simulink model "PID_IdleSpeed"  (R2023b)
settings: Solver=ode15s  StartTime=0.0  StopTime=10  RelTol=1e-3
values from neighbouring files (symbols this model uses):
  DUM = cell2mat(DUM)    [PID_IdleSpeedCode.m]
  NUM = cell2mat(NUM)    [PID_IdleSpeedCode.m]
  Ts = 0.0001    [PID_RL_Tuner.m]
undefined symbols (not defined in the file or in its folder): DiscIntNeverNeededParam
libraries: deeplib x3, slpidlib x2, rllib x2, simulink x2
settings Model: Creator=mrmal  LastModifiedBy=rabia
settings SolverCC: AlgebraicLoopSolver=TrustRegion
settings DebuggingCC: UnconnectedInputMsg=warning  UnconnectedOutputMsg=warning  UnconnectedLineMsg=warning
settings ModelReferenceCC: EnableRefExpFcnMdlSchedulingChecks=on

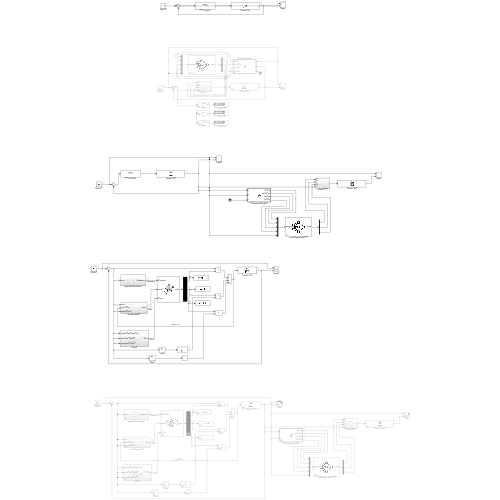
[thumbnail: Simulink's stored preview of the top-level diagram]
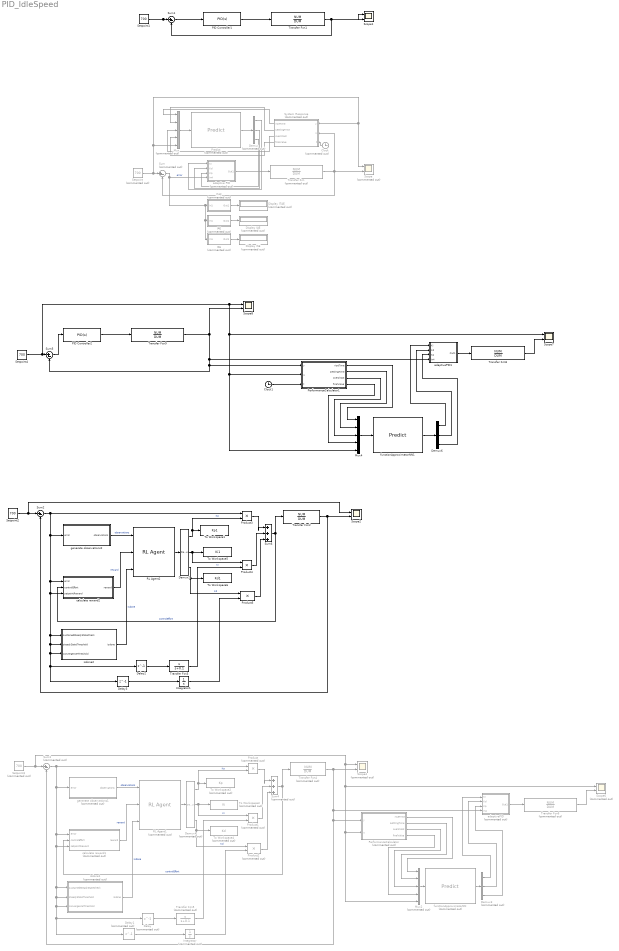
== system PID_IdleSpeed ==
  Clock : Clock  Commented=on
  Clock1 : Clock
  Delay : Delay  Commented=on  DelayLength=1  InitialCondition=0
  Delay1 : Delay  Commented=on  DelayLength=1  InitialCondition=0
  Delay2 : Delay  DelayLength=1  InitialCondition=0
  Delay3 : Delay  DelayLength=1  InitialCondition=0
  Demux : Demux  Commented=on  Outputs=3
  Demux2 : Demux  Outputs=3
  Demux3 : Demux  Commented=on  Outputs=3
  Demux4 : Demux  Commented=on  Outputs=3
  Demux6 : Demux  Outputs=3
  Display IAE : Display  Commented=on
  Display ISE : Display  Commented=on
  Display ITAE : Display  Commented=on
  IAE : Subsystem  Commented=on
      mask help:
      | IAE performacne index
      |
      | output = int |input| dt
      mask Display:
      | disp('IAE')
      | port_label('input',1,'e')
      | port_label('output',1,'iae')
  ISE : Subsystem  Commented=on
      mask help:
      | ISE performance index
      |
      | output = int (input)^2 dt
      mask Display:
      | disp('ISE')
      | port_label('input',1,'e')
      | port_label('output',1,'ise')
  ITAE : Subsystem  Commented=on
      mask help:
      | ITAE performance index
      |
      | output = int t|input| dt
      mask Display:
      | disp('ITAE')
      | port_label('input',1,'e')
      | port_label('output',1,'itae')
  Integrator : Integrator  Commented=on
  Integrator1 : Integrator
  Mux : Mux  Commented=on  Inputs=5
  Mux2 : Mux  Commented=on  Inputs=5
  Mux4 : Mux  Inputs=5
  PID Controller1 : slpidlib/PID Controller  Controller=PID  Form=Parallel  TimeDomain=Continuous-time  UseExternalTs=off  SampleTime=-1  IntegratorMethod=Forward Euler  FilterMethod=Forward Euler  ControllerParametersSource=internal  P=0.1  I=1  UseKiTs=off  D=0.001  N=54.2037558026899  UseFilter=on  TunerSelectOption=Transfer Function Based (PID Tuner App)  InitialConditionSource=internal  InitialConditionForIntegrator=0  InitialConditionForFilter=0  DifferentiatorICPrevScaledInput=0  ExternalReset=none  TrackingMode=off  Kt=1  LimitOutput=off  SatLimitsSource=internal  UpperSaturationLimit=inf  LowerSaturationLimit=-inf  LinearizeAsGain=on  AntiWindupMode=none  Kb=1  LimitIntegrator=off  UpperIntegratorSaturationLimit=inf  LowerIntegratorSaturationLimit=-inf  POutMin=[]  POutMax=[]  IOutMin=[]  IOutMax=[]  DOutMin=[]  DOutMax=[]  NOutMin=[]  NOutMax=[]  SumOutMin=[]  SumOutMax=[]  SaturationOutMin=[]  SaturationOutMax=[]  PParamMin=[]  PParamMax=[]  IParamMin=[]  IParamMax=[]  DParamMin=[]  DParamMax=[]  NParamMin=[]  NParamMax=[]  KbParamMin=[]  KbParamMax=[]  KtParamMin=[]  KtParamMax=[]  KbOutMin=[]  KbOutMax=[]  KtOutMin=[]  KtOutMax=[]  IntegratorOutMin=[]  IntegratorOutMax=[]  FilterOutMin=[]  FilterOutMax=[]  SumI1OutMin=[]  SumI1OutMax=[]  SumI2OutMin=[]  SumI2OutMax=[]  SumI3OutMin=[]  SumI3OutMax=[]  SumI4OutMin=[]  SumI4OutMax=[]  SumDOutMin=[]  SumDOutMax=[]  DifferentiatorOutMin=[]  DifferentiatorOutMax=[]  FilterDiffOutCoefMin=[]  FilterDiffOutCoefMax=[]  ReciprocalOutMin=[]  ReciprocalOutMax=[]  SumDenOutMin=[]  SumDenOutMax=[]  SumNumOutMin=[]  SumNumOutMax=[]  DivideOutMin=[]  DivideOutMax=[]  UdiffTsProdOutMin=[]  UdiffTsProdOutMax=[]  NTsProdOutMin=[]  NTsProdOutMax=[]  UintegralTsProdOutMin=[]  UintegralTsProdOutMax=[]  UngainTsProdOutMin=[]  UngainTsProdOutMax=[]  ClampingZeroOutDataTypeStr=Inherit: Inherit via back propagation  ClampingZeroOutMin=[]  ClampingZeroOutMax=[]  FilterDenConstantOutDataTypeStr=Inherit: Inherit via back propagation  FilterDenConstantOutMin=[]  FilterDenConstantOutMax=[]  PCopyOutDataTypeStr=Inherit: Inherit via back propagation  PCopyOutMin=[]  PCopyOutMax=[]  NCopyOutDataTypeStr=Inherit: Inherit via back propagation  NCopyOutMin=[]  NCopyOutMax=[]  IntegratorContinuousStateAttributes=''  IntegratorStateMustResolveToSignalObject=off  IntegratorRTWStateStorageClass=Auto  FilterContinuousStateAttributes=''  FilterStateMustResolveToSignalObject=off  FilterRTWStateStorageClass=Auto  ParallelPVariant=InternalParameters  IdealPVariant=Disabled  IVariant=InternalParameters  DVariant=InternalParameters  IntegratorVariant=Continuous  SatVariant=Disabled  AWVariant=Passthrough  PCopyVariant=Disabled  TRVariant=Disabled  FdbkBlocksVariant=Forward  IdealPFdbkVariant=Disabled  SatFdbkVariant=Disabled  DerivativeFilterVariant=ContFilter  NVariant=InternalParameters  NCopyVariant=Disabled  FilterICVariant=InternalICsFilter  IntegratorICVariant=InternalICs  ExternalResetVariant=Disabled  TRSumVariant=Passthrough  SumFdbkVariant=Disabled  SumVariant=Sum_PID  TsampFilterVariant=InternalTs  TsampNgainVariant=Passthrough  TsampIntegralVariant=Disabled_SignalSpec  ExternalSaturationOutDataTypeStr=Inherit: Same as second input
  PID Controller2 : slpidlib/PID Controller  Controller=PID  Form=Parallel  TimeDomain=Continuous-time  UseExternalTs=off  SampleTime=-1  IntegratorMethod=Forward Euler  FilterMethod=Forward Euler  ControllerParametersSource=internal  P=0.1  I=1  UseKiTs=off  D=0.001  N=54.2037558026899  UseFilter=on  TunerSelectOption=Transfer Function Based (PID Tuner App)  InitialConditionSource=internal  InitialConditionForIntegrator=0  InitialConditionForFilter=0  DifferentiatorICPrevScaledInput=0  ExternalReset=none  TrackingMode=off  Kt=1  LimitOutput=off  SatLimitsSource=internal  UpperSaturationLimit=inf  LowerSaturationLimit=-inf  LinearizeAsGain=on  AntiWindupMode=none  Kb=1  LimitIntegrator=off  UpperIntegratorSaturationLimit=inf  LowerIntegratorSaturationLimit=-inf  POutMin=[]  POutMax=[]  IOutMin=[]  IOutMax=[]  DOutMin=[]  DOutMax=[]  NOutMin=[]  NOutMax=[]  SumOutMin=[]  SumOutMax=[]  SaturationOutMin=[]  SaturationOutMax=[]  PParamMin=[]  PParamMax=[]  IParamMin=[]  IParamMax=[]  DParamMin=[]  DParamMax=[]  NParamMin=[]  NParamMax=[]  KbParamMin=[]  KbParamMax=[]  KtParamMin=[]  KtParamMax=[]  KbOutMin=[]  KbOutMax=[]  KtOutMin=[]  KtOutMax=[]  IntegratorOutMin=[]  IntegratorOutMax=[]  FilterOutMin=[]  FilterOutMax=[]  SumI1OutMin=[]  SumI1OutMax=[]  SumI2OutMin=[]  SumI2OutMax=[]  SumI3OutMin=[]  SumI3OutMax=[]  SumI4OutMin=[]  SumI4OutMax=[]  SumDOutMin=[]  SumDOutMax=[]  DifferentiatorOutMin=[]  DifferentiatorOutMax=[]  FilterDiffOutCoefMin=[]  FilterDiffOutCoefMax=[]  ReciprocalOutMin=[]  ReciprocalOutMax=[]  SumDenOutMin=[]  SumDenOutMax=[]  SumNumOutMin=[]  SumNumOutMax=[]  DivideOutMin=[]  DivideOutMax=[]  UdiffTsProdOutMin=[]  UdiffTsProdOutMax=[]  NTsProdOutMin=[]  NTsProdOutMax=[]  UintegralTsProdOutMin=[]  UintegralTsProdOutMax=[]  UngainTsProdOutMin=[]  UngainTsProdOutMax=[]  ClampingZeroOutDataTypeStr=Inherit: Inherit via back propagation  ClampingZeroOutMin=[]  ClampingZeroOutMax=[]  FilterDenConstantOutDataTypeStr=Inherit: Inherit via back propagation  FilterDenConstantOutMin=[]  FilterDenConstantOutMax=[]  PCopyOutDataTypeStr=Inherit: Inherit via back propagation  PCopyOutMin=[]  PCopyOutMax=[]  NCopyOutDataTypeStr=Inherit: Inherit via back propagation  NCopyOutMin=[]  NCopyOutMax=[]  IntegratorContinuousStateAttributes=''  IntegratorStateMustResolveToSignalObject=off  IntegratorRTWStateStorageClass=Auto  FilterContinuousStateAttributes=''  FilterStateMustResolveToSignalObject=off  FilterRTWStateStorageClass=Auto  ParallelPVariant=InternalParameters  IdealPVariant=Disabled  IVariant=InternalParameters  DVariant=InternalParameters  IntegratorVariant=Continuous  SatVariant=Disabled  AWVariant=Passthrough  PCopyVariant=Disabled  TRVariant=Disabled  FdbkBlocksVariant=Forward  IdealPFdbkVariant=Disabled  SatFdbkVariant=Disabled  DerivativeFilterVariant=ContFilter  NVariant=InternalParameters  NCopyVariant=Disabled  FilterICVariant=InternalICsFilter  IntegratorICVariant=InternalICs  ExternalResetVariant=Disabled  TRSumVariant=Passthrough  SumFdbkVariant=Disabled  SumVariant=Sum_PID  TsampFilterVariant=InternalTs  TsampNgainVariant=Passthrough  TsampIntegralVariant=Disabled_SignalSpec  ExternalSaturationOutDataTypeStr=Inherit: Same as second input
  PerformanceCalculator : MATLAB Function  Commented=on  TreatAsAtomicUnit=on
  PerformanceCalculator1 : MATLAB Function  TreatAsAtomicUnit=on
  Predict : deeplib/Predict  Commented=on  Network=Network from MAT-file  NetworkFunction=squeezenet  NetworkFilePath=/Users/rabia/Downloads/PID_EngineIdle_Speed/trainedNet.mat  MiniBatchSize=128  InputDataFormats={'',''}  Predictions=on  Activations={}  ForceInterpretedSim=off  EnableDLNetwork=on
  Product : Product  Commented=on
  Product1 : Product  Commented=on
  Product2 : Product  Commented=on
  Product3 : Product
  Product4 : Product
  Product5 : Product
  RL Agent1 : rllib/RL Agent  Commented=on  Agent=agent  ExternalActionAsInput=off  ProvideLastAction=off  ProvideCumRwd=off  TreatAsDirectFeedthrough=on  UseStrictObservationDataTypes=off
  RL Agent2 : rllib/RL Agent  Agent=agent  ExternalActionAsInput=off  ProvideLastAction=off  ProvideCumRwd=off  TreatAsDirectFeedthrough=on  UseStrictObservationDataTypes=off
  Scope : Scope  Commented=on  NumInputPorts=2
  Scope{1..2,7..8} (4 alike) : Scope  NumInputPorts=2
  Scope4 : Scope  Commented=on  NumInputPorts=2
  Scope6 : Scope  Commented=on  NumInputPorts=2
  Setpoint : Constant  Commented=on  Value=700
  Setpoint1 : Constant  Value=700
  Setpoint2 : Constant  Value=700
  Setpoint3 : Constant  Commented=on  Value=700
  Setpoint4 : Constant  Value=700
  Sum : Sum  Commented=on  Inputs=|+-
  Sum1 : Sum  Inputs=|+-
  Sum2 : Sum  Inputs=|+-
  Sum3 : Sum  Commented=on  Inputs=|+-
  Sum4 : Sum  Commented=on  Inputs=|+++
  Sum5 : Sum  Inputs=|+-
  Sum6 : Sum  Inputs=|+++
  System Response : MATLAB Function  Commented=on  TreatAsAtomicUnit=on
  To Workspace1 : ToWorkspace  VariableName=Kp1  SaveFormat=Structure With Time  SampleTime=-1
  To Workspace2 : ToWorkspace  Commented=on  VariableName=Kp  SaveFormat=Structure With Time  SampleTime=-1
  To Workspace3 : ToWorkspace  Commented=on  VariableName=Ki  SaveFormat=Structure With Time  SampleTime=-1
  To Workspace4 : ToWorkspace  Commented=on  VariableName=Kd  SaveFormat=Structure With Time  SampleTime=-1
  To Workspace5 : ToWorkspace  VariableName=Ki1  SaveFormat=Structure With Time  SampleTime=-1
  To Workspace6 : ToWorkspace  VariableName=Kd1  SaveFormat=Structure With Time  SampleTime=-1
  Transfer Fcn : TransferFcn  Commented=on  Numerator=NUM  Denominator=DUM
  Transfer Fcn{1..2,8..9} (4 alike) : TransferFcn  Numerator=NUM  Denominator=DUM
  Transfer Fcn3 : TransferFcn  Numerator=[1, 0]  Denominator=[1, 0.1]
  Transfer Fcn4 : TransferFcn  Commented=on  Numerator=NUM  Denominator=DUM
  Transfer Fcn5 : TransferFcn  Commented=on  Numerator=[1, 0]  Denominator=[1, 0.1]
  Transfer Fcn6 : TransferFcn  Commented=on  Numerator=NUM  Denominator=DUM
  adaptive PID : Subsystem  Commented=on
  adaptivePID : Subsystem  Commented=on
  adaptivePID1 : Subsystem
  calculate reward1 : Subsystem  Commented=on
  calculate reward2 : Subsystem
  functionApproximatorNN : deeplib/Predict  Commented=on  Network=Network from MAT-file  NetworkFunction=squeezenet  NetworkFilePath=/Users/rabia/Downloads/PID_EngineIdle_Speed/trainedNet.mat  MiniBatchSize=128  InputDataFormats={'',''}  Predictions=on  Activations={}  ForceInterpretedSim=off  EnableDLNetwork=on
  functionApproximatorNN1 : deeplib/Predict  Network=Network from MAT-file  NetworkFunction=squeezenet  NetworkFilePath=/Users/rabia/Downloads/PID_EngineIdle_Speed/trainedNet.mat  MiniBatchSize=128  InputDataFormats={'',''}  Predictions=on  Activations={}  ForceInterpretedSim=off  EnableDLNetwork=on
  generate observations1 : Subsystem  Commented=on
  generate observations2 : Subsystem
  isdone1 : Subsystem  Commented=on
  isdone2 : Subsystem
  wires:
  adaptive PID/1(Out1) -> Transfer Fcn/1
  Setpoint/1 -> Sum/1, System Response/1(y), Scope/1, Mux/5
  Transfer Fcn/1 -> Sum/2, Scope/2, System Response/2(u)
  PID Controller1/1 -> Transfer Fcn1/1
  Setpoint1/1 -> Scope1/1, Sum1/1
  Transfer Fcn1/1 -> Sum1/2, Scope1/2
  Sum1/1 -> PID Controller1/1
  Clock/1 -> System Response/3(t)
  ITAE/1(Out1) -> Display ITAE/1
  Sum/1 -> ISE/1(In1), IAE/1(In1), ITAE/1(In1), adaptive PID/4(In4)  "error"
  ISE/1(Out1) -> Display ISE/1
  IAE/1(Out1) -> Display IAE/1
  Predict/1 -> Demux/1
  Mux/1 -> Predict/1
  System Response/4(finalValue) -> Mux/4
  System Response/3(overshoot) -> Mux/3
  System Response/2(settlingTime) -> Mux/2
  System Response/1(riseTime) -> Mux/1
  Demux/3 -> adaptive PID/3(Kp)
  Demux/2 -> adaptive PID/2(Kd)
  Demux/1 -> adaptive PID/1(Ki)
  generate observations1/1(observations) -> RL Agent1/1  "observations"
  calculate reward1/1(reward) -> RL Agent1/2  "reward"
  isdone1/1(isdone) -> RL Agent1/3  "isdone"
  Product/1 -> Sum4/1
  Transfer Fcn5/1 -> Product1/2
  Sum3/1 -> Delay1/1, Delay/1, isdone1/3(convergenceThreshold), isdone1/2(steadyStateThreshold), isdone1/1(sustainedSteadyStateCheck), calculate reward1/3(setpointReward), calculate reward1/1(error), generate observations1/1(error), Product/1
  Product1/1 -> Sum4/2
  Demux4/1 -> To Workspace2/1, Product/2  "Kp"
  Integrator/1 -> Product2/2
  Demux4/3 -> To Workspace4/1, Product2/1  "Kd"
  Demux4/2 -> Product1/1, To Workspace3/1  "Ki"
  Product2/1 -> Sum4/3
  RL Agent1/1 -> Demux4/1
  Sum4/1 -> calculate reward1/2(controlEffort), Transfer Fcn4/1  "controlEffort"
  Delay/1 -> Transfer Fcn5/1
  Delay1/1 -> Integrator/1
  Transfer Fcn4/1 -> Scope4/2, PerformanceCalculator/1(y), Sum3/2, adaptivePID/4(In4)
  Demux3/2 -> adaptivePID/2(Kd)
  Setpoint3/1 -> PerformanceCalculator/2(u), Mux2/5, Scope6/1, Scope4/1, Sum3/1
  Mux2/1 -> functionApproximatorNN/1
  PerformanceCalculator/3(overshoot) -> Mux2/3
  functionApproximatorNN/1 -> Demux3/1
  PerformanceCalculator/1(riseTime) -> Mux2/1
  Transfer Fcn6/1 -> Scope6/2
  Demux3/3 -> adaptivePID/3(Kp)
  PerformanceCalculator/2(settlingTime) -> Mux2/2
  Demux3/1 -> adaptivePID/1(Ki)
  adaptivePID/1(Out1) -> Transfer Fcn6/1
  PerformanceCalculator/4(finalValue) -> Mux2/4
  Setpoint4/1 -> Mux4/5, PerformanceCalculator1/2(u), Scope7/1, Scope8/1, Sum5/1
  Demux6/1 -> adaptivePID1/1(Ki)
  Transfer Fcn9/1 -> Sum5/2, PerformanceCalculator1/1(y), adaptivePID1/4(In4), Scope8/2
  PerformanceCalculator1/1(riseTime) -> Mux4/1
  functionApproximatorNN1/1 -> Demux6/1
  PerformanceCalculator1/2(settlingTime) -> Mux4/2
  Mux4/1 -> functionApproximatorNN1/1
  Transfer Fcn8/1 -> Scope7/2
  PerformanceCalculator1/3(overshoot) -> Mux4/3
  PerformanceCalculator1/4(finalValue) -> Mux4/4
  Demux6/3 -> adaptivePID1/3(Kp)
  Demux6/2 -> adaptivePID1/2(Kd)
  adaptivePID1/1(Out1) -> Transfer Fcn8/1
  Sum5/1 -> PID Controller2/1
  PID Controller2/1 -> Transfer Fcn9/1
  Clock1/1 -> PerformanceCalculator1/3(t)
  Sum6/1 -> calculate reward2/2(controlEffort), Transfer Fcn2/1  "controlEffort"
  generate observations2/1(observations) -> RL Agent2/1  "observations"
  Product4/1 -> Sum6/2
  Integrator1/1 -> Product5/2
  Demux2/2 -> Product4/1, To Workspace5/1  "Ki"
  Demux2/1 -> To Workspace1/1, Product3/2  "Kp"
  Transfer Fcn3/1 -> Product4/2
  Transfer Fcn2/1 -> Scope2/2, Sum2/2
  Product5/1 -> Sum6/3
  Delay2/1 -> Transfer Fcn3/1
  isdone2/1(isdone) -> RL Agent2/3  "isdone"
  Product3/1 -> Sum6/1
  Demux2/3 -> To Workspace6/1, Product5/1  "Kd"
  Delay3/1 -> Integrator1/1
  Setpoint2/1 -> Scope2/1, Sum2/1
  RL Agent2/1 -> Demux2/1
  Sum2/1 -> Delay3/1, Delay2/1, isdone2/3(convergenceThreshold), isdone2/2(steadyStateThreshold), isdone2/1(sustainedSteadyStateCheck), calculate reward2/3(setpointReward), calculate reward2/1(error), generate observations2/1(error), Product3/1
  calculate reward2/1(reward) -> RL Agent2/2  "reward"

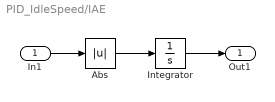
== system PID_IdleSpeed/IAE ==
  In1 : Inport
  Abs : Abs  SaturateOnIntegerOverflow=off
  Integrator : Integrator
  Out1 : Outport
  wires:
  In1/1 -> Abs/1
  Integrator/1 -> Out1/1
  Abs/1 -> Integrator/1

== system PID_IdleSpeed/ISE ==
  In1 : Inport
  Integrator : Integrator
  Math Function : Math  Operator=square  SignedPower=on
  Out1 : Outport
  wires:
  Math Function/1 -> Integrator/1
  Integrator/1 -> Out1/1
  In1/1 -> Math Function/1

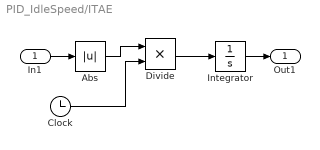
== system PID_IdleSpeed/ITAE ==
  In1 : Inport
  Abs : Abs  SaturateOnIntegerOverflow=off
  Clock : Clock
  Divide : Product  Inputs=**
  Integrator : Integrator
  Out1 : Outport
  wires:
  Integrator/1 -> Out1/1
  In1/1 -> Abs/1
  Divide/1 -> Integrator/1
  Abs/1 -> Divide/1
  Clock/1 -> Divide/2

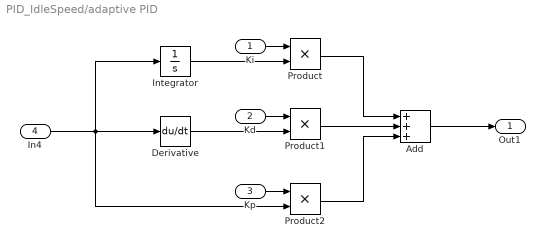
== system PID_IdleSpeed/adaptive PID ==
  Ki : Inport
  Kd : Inport  Port=2
  Kp : Inport  Port=3
  In4 : Inport  Port=4
  Add : Sum  Inputs=+++
  Derivative : Derivative
  Integrator : Integrator
  Product : Product
  Product1 : Product
  Product2 : Product
  Out1 : Outport
  wires:
  Integrator/1 -> Product/2
  Kp/1 -> Product2/1
  In4/1 -> Product2/2, Derivative/1, Integrator/1
  Product/1 -> Add/1
  Product1/1 -> Add/2
  Product2/1 -> Add/3
  Derivative/1 -> Product1/2
  Ki/1 -> Product/1
  Kd/1 -> Product1/1
  Add/1 -> Out1/1

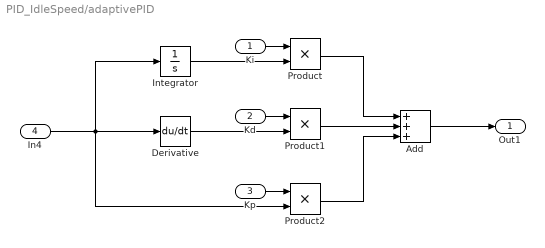
== system PID_IdleSpeed/adaptivePID ==
  Ki : Inport
  Kd : Inport  Port=2
  Kp : Inport  Port=3
  In4 : Inport  Port=4
  Add : Sum  Inputs=+++
  Derivative : Derivative
  Integrator : Integrator
  Product : Product
  Product1 : Product
  Product2 : Product
  Out1 : Outport
  wires:
  Integrator/1 -> Product/2
  Kp/1 -> Product2/1
  In4/1 -> Product2/2, Derivative/1, Integrator/1
  Product/1 -> Add/1
  Product1/1 -> Add/2
  Product2/1 -> Add/3
  Derivative/1 -> Product1/2
  Ki/1 -> Product/1
  Kd/1 -> Product1/1
  Add/1 -> Out1/1

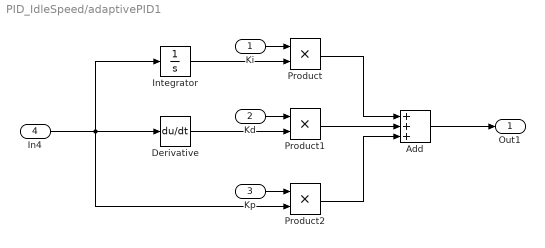
== system PID_IdleSpeed/adaptivePID1 ==
  Ki : Inport
  Kd : Inport  Port=2
  Kp : Inport  Port=3
  In4 : Inport  Port=4
  Add : Sum  Inputs=+++
  Derivative : Derivative
  Integrator : Integrator
  Product : Product
  Product1 : Product
  Product2 : Product
  Out1 : Outport
  wires:
  Integrator/1 -> Product/2
  Kp/1 -> Product2/1
  In4/1 -> Product2/2, Derivative/1, Integrator/1
  Product/1 -> Add/1
  Product1/1 -> Add/2
  Product2/1 -> Add/3
  Derivative/1 -> Product1/2
  Ki/1 -> Product/1
  Kd/1 -> Product1/1
  Add/1 -> Out1/1

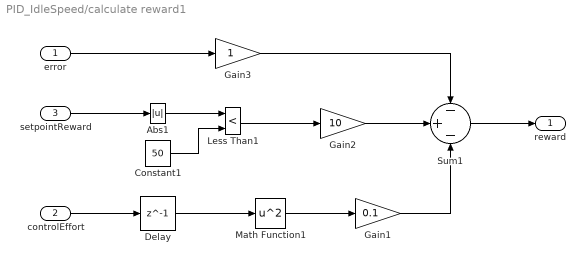
== system PID_IdleSpeed/calculate reward1 ==
  error : Inport
  controlEffort : Inport  Port=2
  setpointReward : Inport  Port=3
  Abs1 : Abs  SaturateOnIntegerOverflow=off
  Constant1 : Constant  Value=50
  Delay : Delay  DelayLength=1  InitialCondition=0
  Gain1 : Gain  Gain=0.1
  Gain2 : Gain  Gain=10
  Gain3 : Gain
  Less Than1 : RelationalOperator  Operator=<  OutDataTypeStr=boolean  RndMeth=Simplest  InputSameDT=off
  Math Function1 : Math  Operator=square
  Sum1 : Sum  Inputs=-+-  OutDataTypeStr=double
  reward : Outport  VectorParamsAs1DForOutWhenUnconnected=off
  wires:
  error/1 -> Gain3/1
  Gain3/1 -> Sum1/1
  Sum1/1 -> reward/1
  Math Function1/1 -> Gain1/1
  Gain1/1 -> Sum1/3
  controlEffort/1 -> Delay/1
  setpointReward/1 -> Abs1/1
  Constant1/1 -> Less Than1/2
  Less Than1/1 -> Gain2/1
  Abs1/1 -> Less Than1/1
  Gain2/1 -> Sum1/2
  Delay/1 -> Math Function1/1

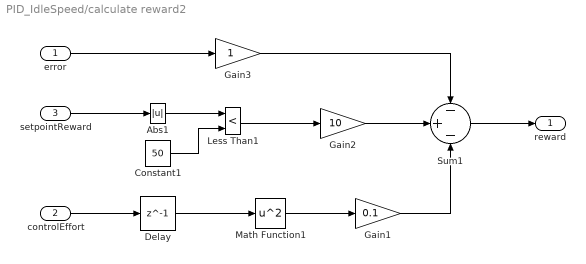
== system PID_IdleSpeed/calculate reward2 ==
  error : Inport
  controlEffort : Inport  Port=2
  setpointReward : Inport  Port=3
  Abs1 : Abs  SaturateOnIntegerOverflow=off
  Constant1 : Constant  Value=50
  Delay : Delay  DelayLength=1  InitialCondition=0
  Gain1 : Gain  Gain=0.1
  Gain2 : Gain  Gain=10
  Gain3 : Gain
  Less Than1 : RelationalOperator  Operator=<  OutDataTypeStr=boolean  RndMeth=Simplest  InputSameDT=off
  Math Function1 : Math  Operator=square
  Sum1 : Sum  Inputs=-+-  OutDataTypeStr=double
  reward : Outport  VectorParamsAs1DForOutWhenUnconnected=off
  wires:
  error/1 -> Gain3/1
  Gain3/1 -> Sum1/1
  Sum1/1 -> reward/1
  Math Function1/1 -> Gain1/1
  Gain1/1 -> Sum1/3
  controlEffort/1 -> Delay/1
  setpointReward/1 -> Abs1/1
  Constant1/1 -> Less Than1/2
  Less Than1/1 -> Gain2/1
  Abs1/1 -> Less Than1/1
  Gain2/1 -> Sum1/2
  Delay/1 -> Math Function1/1

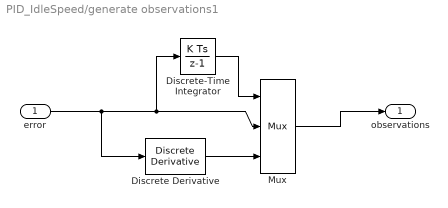
== system PID_IdleSpeed/generate observations1 ==
  error : Inport
  Discrete Derivative : simulink/Discrete/Discrete Derivative  gainval=1.0  ICPrevScaledInput=0.0  OutMin=[]  OutMax=[]  OutDataType=fixdt(1, 16)  OutScaling=2^-10  DoSatur=off
  Discrete-Time Integrator : DiscreteIntegrator  SampleTime=Ts  ICPrevOutput=DiscIntNeverNeededParam  ICPrevScaledInput=DiscIntNeverNeededParam
  Mux : Mux  Inputs=3
  observations : Outport  VectorParamsAs1DForOutWhenUnconnected=off
  wires:
  Discrete-Time Integrator/1 -> Mux/1
  error/1 -> Discrete Derivative/1, Discrete-Time Integrator/1, Mux/2
  Mux/1 -> observations/1
  Discrete Derivative/1 -> Mux/3

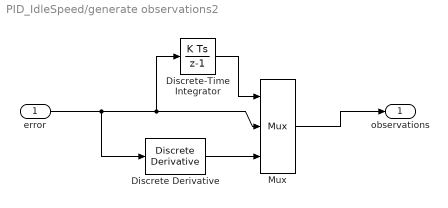
== system PID_IdleSpeed/generate observations2 ==
  error : Inport
  Discrete Derivative : simulink/Discrete/Discrete Derivative  gainval=1.0  ICPrevScaledInput=0.0  OutMin=[]  OutMax=[]  OutDataType=fixdt(1, 16)  OutScaling=2^-10  DoSatur=off
  Discrete-Time Integrator : DiscreteIntegrator  SampleTime=Ts  ICPrevOutput=DiscIntNeverNeededParam  ICPrevScaledInput=DiscIntNeverNeededParam
  Mux : Mux  Inputs=3
  observations : Outport  VectorParamsAs1DForOutWhenUnconnected=off
  wires:
  Discrete-Time Integrator/1 -> Mux/1
  error/1 -> Discrete Derivative/1, Discrete-Time Integrator/1, Mux/2
  Mux/1 -> observations/1
  Discrete Derivative/1 -> Mux/3

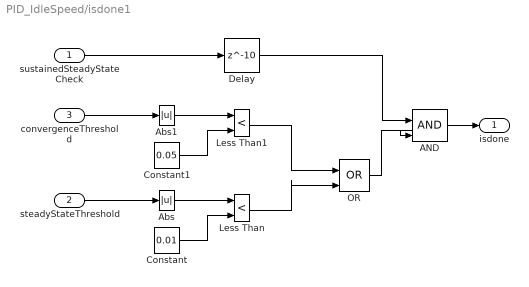
== system PID_IdleSpeed/isdone1 ==
  sustainedSteadyStateCheck : Inport
  steadyStateThreshold : Inport  Port=2
  convergenceThreshold : Inport  Port=3
  AND : Logic  IconShape=distinctive  AllPortsSameDT=off  OutDataTypeStr=boolean
  Abs : Abs  SaturateOnIntegerOverflow=off
  Abs1 : Abs  SaturateOnIntegerOverflow=off
  Constant : Constant  Value=0.01
  Constant1 : Constant  Value=0.05
  Delay : Delay  DelayLength=10  InitialCondition=0
  Less Than : RelationalOperator  Operator=<  OutDataTypeStr=boolean  RndMeth=Simplest  InputSameDT=off
  Less Than1 : RelationalOperator  Operator=<  OutDataTypeStr=boolean  RndMeth=Simplest  InputSameDT=off
  OR : Logic  Operator=OR  IconShape=distinctive  AllPortsSameDT=off  OutDataTypeStr=boolean
  isdone : Outport  VectorParamsAs1DForOutWhenUnconnected=off
  wires:
  steadyStateThreshold/1 -> Abs/1
  sustainedSteadyStateCheck/1 -> Delay/1
  AND/1 -> isdone/1
  Less Than/1 -> OR/2
  Abs/1 -> Less Than/1
  Constant/1 -> Less Than/2
  convergenceThreshold/1 -> Abs1/1
  Less Than1/1 -> OR/1
  Constant1/1 -> Less Than1/2
  Abs1/1 -> Less Than1/1
  Delay/1 -> AND/1
  OR/1 -> AND/2

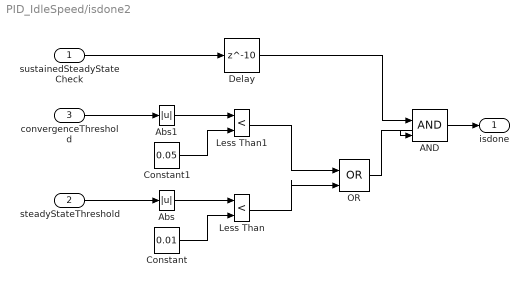
== system PID_IdleSpeed/isdone2 ==
  sustainedSteadyStateCheck : Inport
  steadyStateThreshold : Inport  Port=2
  convergenceThreshold : Inport  Port=3
  AND : Logic  IconShape=distinctive  AllPortsSameDT=off  OutDataTypeStr=boolean
  Abs : Abs  SaturateOnIntegerOverflow=off
  Abs1 : Abs  SaturateOnIntegerOverflow=off
  Constant : Constant  Value=0.01
  Constant1 : Constant  Value=0.05
  Delay : Delay  DelayLength=10  InitialCondition=0
  Less Than : RelationalOperator  Operator=<  OutDataTypeStr=boolean  RndMeth=Simplest  InputSameDT=off
  Less Than1 : RelationalOperator  Operator=<  OutDataTypeStr=boolean  RndMeth=Simplest  InputSameDT=off
  OR : Logic  Operator=OR  IconShape=distinctive  AllPortsSameDT=off  OutDataTypeStr=boolean
  isdone : Outport  VectorParamsAs1DForOutWhenUnconnected=off
  wires:
  steadyStateThreshold/1 -> Abs/1
  sustainedSteadyStateCheck/1 -> Delay/1
  AND/1 -> isdone/1
  Less Than/1 -> OR/2
  Abs/1 -> Less Than/1
  Constant/1 -> Less Than/2
  convergenceThreshold/1 -> Abs1/1
  Less Than1/1 -> OR/1
  Constant1/1 -> Less Than1/2
  Abs1/1 -> Less Than1/1
  Delay/1 -> AND/1
  OR/1 -> AND/2

== matlab function PID_IdleSpeed/System Response ==
  data: y input; u input; riseTime output; t input; settlingTime output; overshoot output; finalValue output
function [riseTime, settlingTime, overshoot, finalValue] = fcn(y, u, t)
    % Persistent variables hold the state of the computation between time steps
    persistent maxVal riseTimeComputed settlingTimeComputed lastValue lastTime tStart overshootComputed
    
    % Initialize persistent variables if empty
    if isempty(riseTimeComputed)
        riseTimeComputed = false;
        settlingTimeComputed = false;
        overshootComputed = false;
        maxVal = 0;
        riseTime = Inf;
        settlingTime = Inf;
        finalValue = 0;
        overshoot = 0;
        lastValue = 0;
        lastTime = 0;
        tStart = t;
    end
    
    % Constants for performance metrics thresholds
    riseThreshold = 0.9 * u; % 90% of the setpoint
    settlingThreshold = 0.02 * u; % 2% of the setpoint
    settleTimeWindow = 1; % Time window to consider for settling
    
    % Check for new max value and overshoot
    if y > maxVal
        maxVal = y;
        if ~overshootComputed && y > u
            overshoot = (y - u) / u * 100; % overshoot in percentage
            overshootComputed = true;
        end
    else
        if ~overshootComputed
            overshoot = 0; % Confirm no overshoot if max value is not exceeded
        end
    end
    
    % Check for rise time
    if ~riseTimeComputed && y >= riseThreshold
        riseTime = t - tStart;
        riseTimeComputed = true;
    elseif ~riseTimeComputed
        riseTime = Inf; % Confirm not computed if threshold is not met
    end
    
    % Check for settling time
    if ~settlingTimeComputed
        if abs(lastValue - u) > settlingThreshold
            lastTime = t;
        elseif t - lastTime >= settleTimeWindow
            settlingTime = lastTime - tStart;
            settlingTimeComputed = true;
        end
    else
        if ~settlingTimeComputed
            settlingTime = Inf; % Confirm not computed if conditions are not met
        end
    end
    
    % Update the last known value
    lastValue = y;
    
    % Assuming the final value is the last value of the output
    finalValue = lastValue;
end

== matlab function PID_IdleSpeed/PerformanceCalculator ==
  data: y input; u input; riseTime output; settlingTime output; overshoot output; finalValue output
function [riseTime, settlingTime, overshoot, finalValue] = fcn(y, u)
    % Persistent variables hold the state of the computation between time steps
    persistent maxVal riseTimeComputed settlingTimeComputed lastValue lastTime tStart overshootComputed
    
    % Initialize persistent variables if empty
    if isempty(riseTimeComputed)
        riseTimeComputed = false;
        settlingTimeComputed = false;
        overshootComputed = false;
        maxVal = 0;
        riseTime = Inf;
        settlingTime = Inf;
        finalValue = 0;
        overshoot = 0;
        lastValue = 0;
        lastTime = 0;
        tStart = t;
    end
    
    % Constants for performance metrics thresholds
    riseThreshold = 0.9 * u; % 90% of the setpoint
    settlingThreshold = 0.02 * u; % 2% of the setpoint
    settleTimeWindow = 1; % Time window to consider for settling
    
    % Check for new max value and overshoot
    if y > maxVal
        maxVal = y;
        if ~overshootComputed && y > u
            overshoot = (y - u) / u * 100; % overshoot in percentage
            overshootComputed = true;
        end
    else
        if ~overshootComputed
            overshoot = 0; % Confirm no overshoot if max value is not exceeded
        end
    end
    
    % Check for rise time
    if ~riseTimeComputed && y >= riseThreshold
        riseTime = t - tStart;
        riseTimeComputed = true;
    elseif ~riseTimeComputed
        riseTime = Inf; % Confirm not computed if threshold is not met
    end
    
    % Check for settling time
    if ~settlingTimeComputed
        if abs(lastValue - u) > settlingThreshold
            lastTime = t;
        elseif t - lastTime >= settleTimeWindow
            settlingTime = lastTime - tStart;
            settlingTimeComputed = true;
        end
    else
        if ~settlingTimeComputed
            settlingTime = Inf; % Confirm not computed if conditions are not met
        end
    end
    
    % Update the last known value
    lastValue = y;
    
    % Assuming the final value is the last value of the output
    finalValue = lastValue;
end

== matlab function PID_IdleSpeed/PerformanceCalculator1 ==
  data: y input; u input; riseTime output; settlingTime output; overshoot output; finalValue output; t input
function [riseTime, settlingTime, overshoot, finalValue] = fcn(y, u, t)
    % Persistent variables hold the state of the computation between time steps
    persistent maxVal riseTimeComputed settlingTimeComputed lastValue lastTime tStart overshootComputed
    
    % Initialize persistent variables if empty
    if isempty(riseTimeComputed)
        riseTimeComputed = false;
        settlingTimeComputed = false;
        overshootComputed = false;
        maxVal = 0;
        riseTime = Inf;
        settlingTime = Inf;
        finalValue = 0;
        overshoot = 0;
        lastValue = 0;
        lastTime = 0;
        tStart = t;
    end
    
    % Constants for performance metrics thresholds
    riseThreshold = 0.9 * u; % 90% of the setpoint
    settlingThreshold = 0.02 * u; % 2% of the setpoint
    settleTimeWindow = 1; % Time window to consider for settling
    
    % Check for new max value and overshoot
    if y > maxVal
        maxVal = y;
        if ~overshootComputed && y > u
            overshoot = (y - u) / u * 100; % overshoot in percentage
            overshootComputed = true;
        end
    else
        if ~overshootComputed
            overshoot = 0; % Confirm no overshoot if max value is not exceeded
        end
    end
    
    % Check for rise time
    if ~riseTimeComputed && y >= riseThreshold
        riseTime = t - tStart;
        riseTimeComputed = true;
    elseif ~riseTimeComputed
        riseTime = Inf; % Confirm not computed if threshold is not met
    end
    
    % Check for settling time
    if ~settlingTimeComputed
        if abs(lastValue - u) > settlingThreshold
            lastTime = t;
        elseif t - lastTime >= settleTimeWindow
            settlingTime = lastTime - tStart;
            settlingTimeComputed = true;
        end
    else
        if ~settlingTimeComputed
            settlingTime = Inf; % Confirm not computed if conditions are not met
        end
    end
    
    % Update the last known value
    lastValue = y;
    
    % Assuming the final value is the last value of the output
    finalValue = lastValue;
end
